simulink model "cv4model"  (R2021a)
settings: Solver=VariableStepAuto  StartTime=0.0  StopTime=600  RelTol=1e-3
values from neighbouring files (symbols this model uses):
  I = ar(:,2) / 6    [cv4.m]    (also in cv4GA.m; cv4_bergman.m; cv4_bergmanGA.m; surove.m = s1.I(4001:end))
  Ib = 12.3165    [afterGA.m]    (also in bergmanGA.m = insuline(1); cv3.m = insuline(1); cv3a.m = insuline(1); cv4.m)
  kI = 0.1645    [afterGA.m]    (also in cv4.m; cv4GA.m = Best(2); cv4_bergman.m; cv4_bergmanGA.m)
  S1b = 1.2528e4    (= 12528)    [afterGA.m]    (also in cv4.m; cv4GA.m; cv4_bergman.m; cv4_bergmanGA.m)
  S2b = S1b    (= 12528)    [afterGA.m]    (also in cv4.m; cv4GA.m; cv4_bergman.m; cv4_bergmanGA.m)
  T = readtable('Dat_IVGTT_RI.csv')    [bergmanGA.m]    (also in cv3.m = readtable('Dat_IVGTT_SN.csv'); cv3a.m; cv4.m = ar(:,1); cv4GA.m = ar(:,1))
  TI = 44.55    [afterGA.m]    (also in cv4.m; cv4GA.m = Best(1); cv4_bergman.m; cv4_bergmanGA.m)
  VI = 138.8    [afterGA.m]    (also in cv4.m; cv4GA.m = Best(3); cv4_bergman.m; cv4_bergmanGA.m)
settings Model: Creator=marko  LastModifiedBy=marko

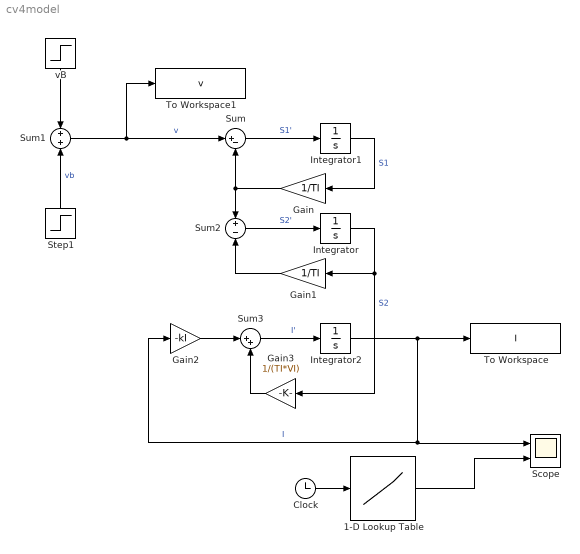
== system cv4model ==
  1-D Lookup Table : Lookup_n-D  NumberOfTableDimensions=1  BreakpointsForDimension1=T  Table=I  InternalRulePriority=Speed  RndMeth=Simplest  InputSameDT=on
  Clock : Clock
  Gain : Gain  Gain=1/TI
  Gain1 : Gain  Gain=1/TI
  Gain2 : Gain  Gain=-kI
  Gain3 : Gain  Gain=1/(TI*VI)
  Integrator : Integrator  InitialCondition=S2b
  Integrator1 : Integrator  InitialCondition=S1b
  Integrator2 : Integrator  InitialCondition=Ib
  Scope : Scope  NumInputPorts=2
  Step1 : Step  Time=0  After=281.218  SampleTime=0
  Sum : Sum  Inputs=|+-
  Sum1 : Sum  Inputs=+|+
  Sum2 : Sum  Inputs=+|-
  Sum3 : Sum  Inputs=|++
  To Workspace : ToWorkspace  VariableName=I  SaveFormat=Timeseries  SampleTime=-1
  To Workspace1 : ToWorkspace  VariableName=v  SaveFormat=Timeseries  SampleTime=-1
  vB : Step  Time=5  Before=40000  After=0  SampleTime=0
  wires:
  Integrator1/1 -> Gain/1  "S1"
  Sum/1 -> Integrator1/1  "S1'"
  Sum1/1 -> To Workspace1/1, Sum/1  "v"
  vB/1 -> Sum1/1
  Step1/1 -> Sum1/2  "vb"
  Integrator/1 -> Gain3/1, Gain1/1  "S2"
  Sum2/1 -> Integrator/1  "S2'"
  Gain/1 -> Sum/2, Sum2/1
  Gain1/1 -> Sum2/2
  Gain3/1 -> Sum3/2
  Sum3/1 -> Integrator2/1  "I'"
  Gain2/1 -> Sum3/1
  Integrator2/1 -> Gain2/1, Scope/1, To Workspace/1  "I"
  Clock/1 -> 1-D Lookup Table/1
  1-D Lookup Table/1 -> Scope/2
